simulink model "Simulation_2_Wall_Follower_v1"  (R2023a)
settings: Solver=ode1  StartTime=0.0  StopTime=inf  RelTol=1e-3
values from neighbouring files (symbols this model uses):
  D = [ D0 D1 D2 D3 D4 ]    [constante.m]    (also in data.mat = [8 8 8 8 8])
  K = [ K0 K1  0 K3 K4 ]    [constante.m]    (also in data.mat = [1.0471975512 0.523598775598 0 -0.523598775598 -1.0471975512)
  L = 5    [constante.m]    (also in data.mat)
  maze = gobjects    [animation.m]    (also in data.mat = [0 0 0 0 0 0 0 0 0 0 0 0 ... (94249 elements, 307x307)]; setup.m = cat(2,maze,add_column))
  number_add = 50    [data.mat]    (also in setup.m)
  S_max = 20    [constante.m]    (also in data.mat)
  S_sens = 0.1    [constante.m]    (also in data.mat)
  size_map = 307    [data.mat]    (also in setup.m = length(maze))
  Theta_d = -1.57079632679    [data.mat]
  Vd = 0.05    [data.mat]    (also in setup.m)
  Vg = 0.05    [data.mat]    (also in setup.m)
  Xd = 70    [data.mat]
  Yd = 170    [data.mat]
settings Model: Creator=Nas  LastModifiedBy=lespi
settings SolverCC: AlgebraicLoopSolver=TrustRegion
settings DataIOCC: ReturnWorkspaceOutputs=off
settings DebuggingCC: UnconnectedInputMsg=warning  UnconnectedOutputMsg=warning  UnconnectedLineMsg=warning  ArithmeticOperatorsInVariantConditions=warning
settings ModelReferenceCC: EnableRefExpFcnMdlSchedulingChecks=on
settings SFSimCC: SimUseLocalCustomCode=off  CustomCodeUndefinedFunction=UseInterfaceOnly
settings RTWCC: RTWUseLocalCustomCode=off

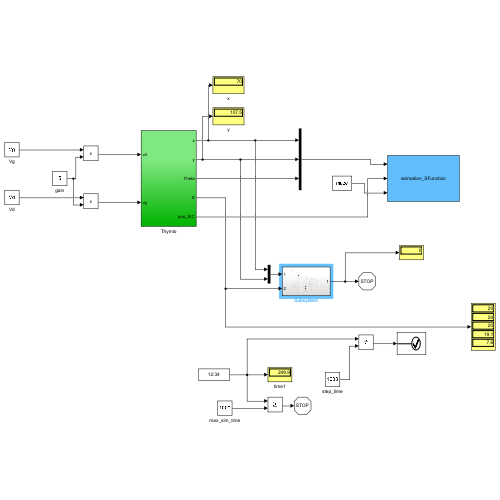
[thumbnail: Simulink's stored preview of the top-level diagram]
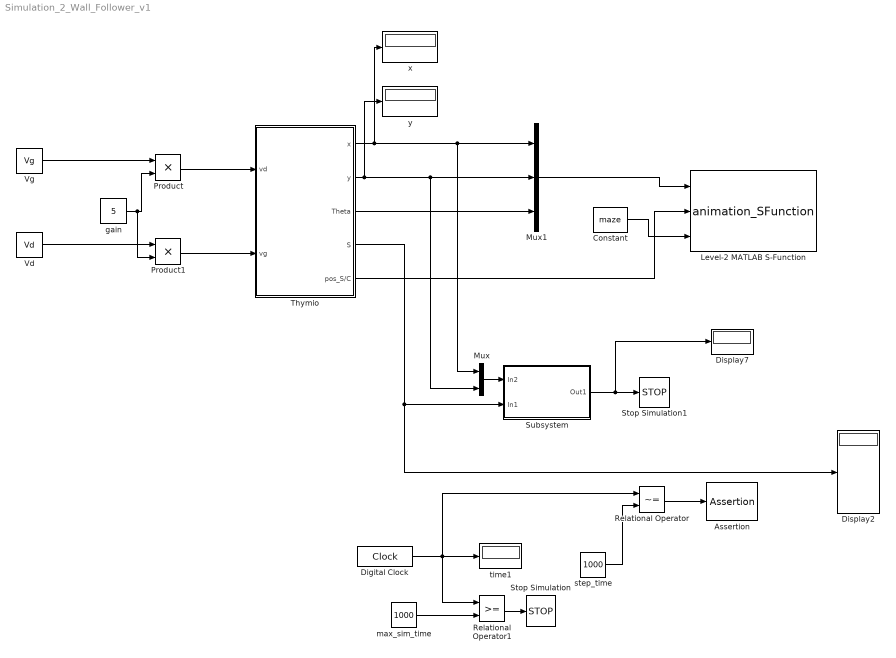
== system Simulation_2_Wall_Follower_v1 ==
  Assertion : Assertion  AssertionFailFcn=set_param(bdroot,'SimulationCommand','pause')  StopWhenAssertionFail=off
  Constant : Constant  Value=maze
  Digital Clock : DigitalClock  SampleTime=0.1
  Display2 : Display
  Display7 : Display
  Level-2 MATLAB S-Function : M-S-Function  FunctionName=animation_SFunction
  Mux : Mux  Inputs=2
  Mux1 : Mux  Inputs=3
  Product : Product
  Product1 : Product
  Relational Operator : RelationalOperator  Operator=~=  OutDataTypeStr=boolean  RndMeth=Simplest  InputSameDT=off
  Relational Operator1 : RelationalOperator  OutDataTypeStr=boolean  RndMeth=Simplest  InputSameDT=off
  Stop Simulation : Stop
  Stop Simulation1 : Stop
  Subsystem : Subsystem
  Thymio : Subsystem
  Vd : Constant  Value=Vd
  Vg : Constant  Value=Vg
  gain : Constant  Value=5
  max_sim_time : Constant  Value=1000
  step_time : Constant  Value=1000
  time1 : Display
  x : Display
  y : Display
  wires:
  Vd/1 -> Product1/1
  Vg/1 -> Product/1
  Mux1/1 -> Level-2 MATLAB S-Function/1
  Thymio/5(pos_S/C) -> Level-2 MATLAB S-Function/2
  Thymio/1(x) -> x/1, Mux/1, Mux1/1
  Mux/1 -> Subsystem/1(In2)
  Thymio/3(Theta) -> Mux1/3
  Thymio/2(y) -> Mux/2, Mux1/2, y/1
  Thymio/4(S) -> Display2/1, Subsystem/2(In1)
  Constant/1 -> Level-2 MATLAB S-Function/3
  gain/1 -> Product1/2, Product/2
  Product1/1 -> Thymio/2(vg)
  Product/1 -> Thymio/1(vd)
  step_time/1 -> Relational Operator/2
  Relational Operator/1 -> Assertion/1
  Digital Clock/1 -> time1/1, Relational Operator1/1, Relational Operator/1
  max_sim_time/1 -> Relational Operator1/2
  Relational Operator1/1 -> Stop Simulation/1
  Subsystem/1(Out1) -> Display7/1, Stop Simulation1/1

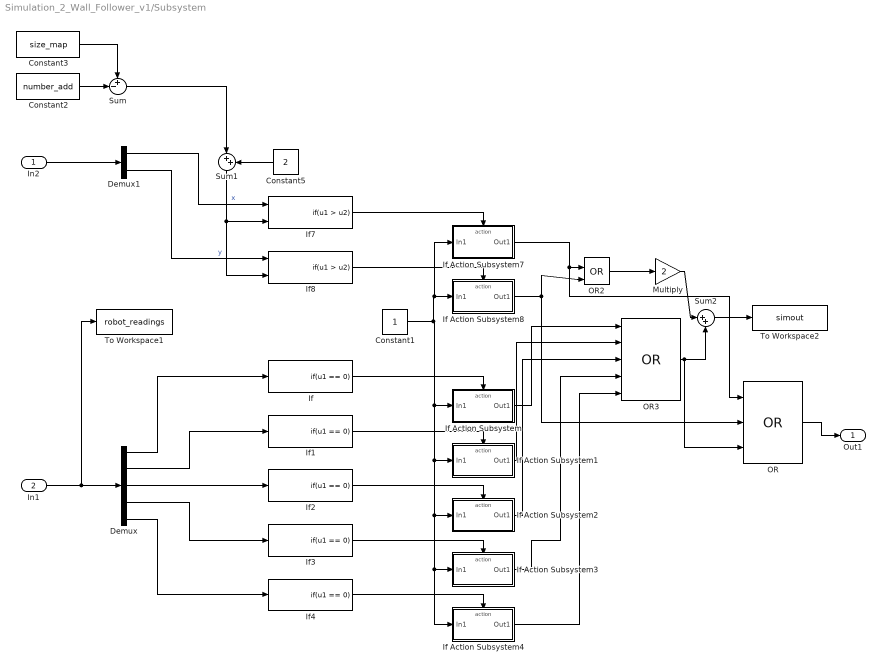
== system Simulation_2_Wall_Follower_v1/Subsystem ==
  In2 : Inport
  In1 : Inport  Port=2
  Constant1 : Constant
  Constant2 : Constant  Value=number_add
  Constant3 : Constant  Value=size_map
  Constant5 : Constant  Value=2
  Demux : Demux  Outputs=5
  Demux1 : Demux  Outputs=2
  If{,1..4} (5 alike) : If  IfExpression=u1 == 0  ShowElse=off
  If Action Subsystem : Subsystem  TreatAsAtomicUnit=on
  If Action Subsystem1 : Subsystem  TreatAsAtomicUnit=on
  If Action Subsystem2 : Subsystem  TreatAsAtomicUnit=on
  If Action Subsystem3 : Subsystem  TreatAsAtomicUnit=on
  If Action Subsystem4 : Subsystem  TreatAsAtomicUnit=on
  If Action Subsystem7 : Subsystem  TreatAsAtomicUnit=on
  If Action Subsystem8 : Subsystem  TreatAsAtomicUnit=on
  If7 : If  NumInputs=2  IfExpression=u1 > u2  ShowElse=off
  If8 : If  NumInputs=2  IfExpression=u1 > u2  ShowElse=off
  Multiply : Gain  Gain=2
  OR : Logic  Operator=OR  Inputs=3  IconShape=distinctive  AllPortsSameDT=off  OutDataTypeStr=boolean
  OR2 : Logic  Operator=OR  IconShape=distinctive  AllPortsSameDT=off  OutDataTypeStr=boolean
  OR3 : Logic  Operator=OR  Inputs=5  IconShape=distinctive  AllPortsSameDT=off  OutDataTypeStr=boolean
  Sum : Sum  Inputs=+-|
  Sum1 : Sum  Inputs=|++
  Sum2 : Sum  Inputs=|++
  To Workspace1 : ToWorkspace  VariableName=robot_readings  SaveFormat=Timeseries  SampleTime=-1
      settings: MaxDataPoints=1
  To Workspace2 : ToWorkspace  VariableName=simout  SaveFormat=Timeseries  SampleTime=-1
      settings: MaxDataPoints=1
  Out1 : Outport  VectorParamsAs1DForOutWhenUnconnected=off
  wires:
  Constant1/1 -> If Action Subsystem7/1(In1), If Action Subsystem8/1(In1), If Action Subsystem1/1(In1), If Action Subsystem2/1(In1), If Action Subsystem3/1(In1), If Action Subsystem4/1(In1), If Action Subsystem/1(In1)
  In1/1 -> To Workspace1/1, Demux/1
  Demux/1 -> If/1
  Demux/2 -> If1/1
  Demux/3 -> If2/1
  Demux/4 -> If3/1
  Demux/5 -> If4/1
  If/1 -> If Action Subsystem/Action
  If1/1 -> If Action Subsystem1/Action
  If2/1 -> If Action Subsystem2/Action
  If3/1 -> If Action Subsystem3/Action
  If4/1 -> If Action Subsystem4/Action
  OR/1 -> Out1/1
  In2/1 -> Demux1/1
  Demux1/2 -> If8/1  "y"
  Demux1/1 -> If7/1  "x"
  Constant3/1 -> Sum/1
  Constant2/1 -> Sum/2
  Sum/1 -> Sum1/1
  Sum1/1 -> If7/2, If8/2
  Constant5/1 -> Sum1/2
  If Action Subsystem7/1(Out1) -> OR2/1, OR/1
  If Action Subsystem8/1(Out1) -> OR/2, OR2/2
  If8/1 -> If Action Subsystem8/Action
  If7/1 -> If Action Subsystem7/Action
  If Action Subsystem4/1(Out1) -> OR3/5
  If Action Subsystem3/1(Out1) -> OR3/4
  If Action Subsystem2/1(Out1) -> OR3/3
  If Action Subsystem1/1(Out1) -> OR3/2
  If Action Subsystem/1(Out1) -> OR3/1
  OR2/1 -> Multiply/1
  OR3/1 -> OR/3, Sum2/2
  Multiply/1 -> Sum2/1
  Sum2/1 -> To Workspace2/1

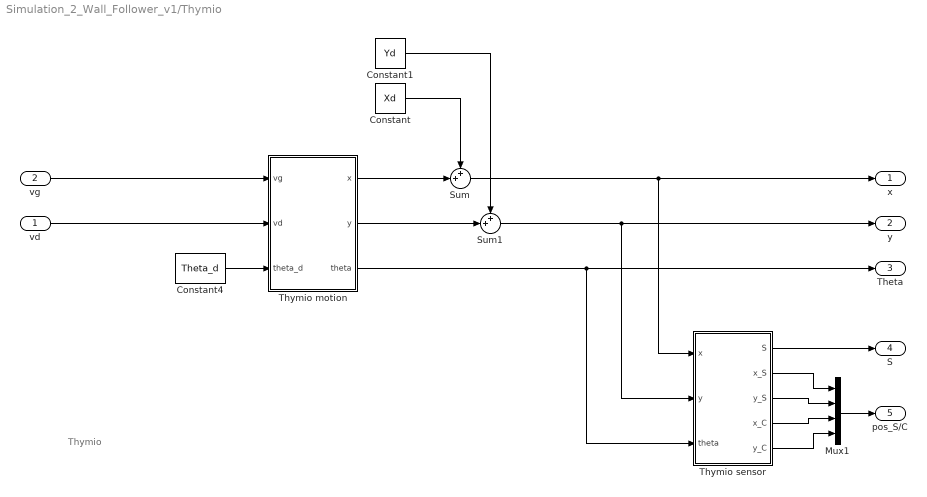
== system Simulation_2_Wall_Follower_v1/Thymio ==
  note: Thymio
  vd : Inport
  vg : Inport  Port=2
  Constant : Constant  Value=Xd
  Constant1 : Constant  Value=Yd
  Constant4 : Constant  Value=Theta_d
  Mux1 : Mux
  Sum : Sum  Inputs=++|
  Sum1 : Sum  Inputs=++|
  Thymio motion : Subsystem
  Thymio sensor : Subsystem
  x : Outport  VectorParamsAs1DForOutWhenUnconnected=off
  y : Outport  Port=2  VectorParamsAs1DForOutWhenUnconnected=off
  Theta : Outport  Port=3  VectorParamsAs1DForOutWhenUnconnected=off
  S : Outport  Port=4  VectorParamsAs1DForOutWhenUnconnected=off
  pos_S/C : Outport  Port=5  VectorParamsAs1DForOutWhenUnconnected=off
  wires:
  Constant4/1 -> Thymio motion/3(theta_d)
  Sum1/1 -> Thymio sensor/2(y), y/1
  Thymio motion/2(y) -> Sum1/2
  Constant/1 -> Sum/1
  Thymio motion/3(theta) -> Thymio sensor/3(theta), Theta/1
  Constant1/1 -> Sum1/1
  Sum/1 -> Thymio sensor/1(x), x/1
  Thymio motion/1(x) -> Sum/2
  vg/1 -> Thymio motion/1(vg)
  vd/1 -> Thymio motion/2(vd)
  Thymio sensor/1(S) -> S/1
  Thymio sensor/2(x_S) -> Mux1/1
  Thymio sensor/3(y_S) -> Mux1/2
  Mux1/1 -> pos_S/C/1
  Thymio sensor/4(x_C) -> Mux1/3
  Thymio sensor/5(y_C) -> Mux1/4

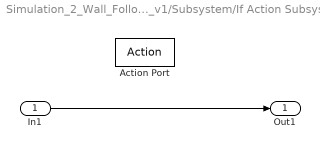
== system Simulation_2_Wall_Follower_v1/Subsystem/If Action Subsystem ==
  In1 : Inport
  Action Port : ActionPort  ActionPortLabel=if(u1 == 0)
  Out1 : Outport  VectorParamsAs1DForOutWhenUnconnected=off
  wires:
  In1/1 -> Out1/1

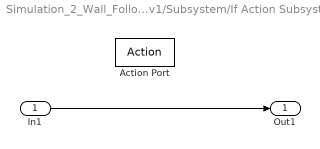
== system Simulation_2_Wall_Follower_v1/Subsystem/If Action Subsystem1 ==
  In1 : Inport
  Action Port : ActionPort  ActionPortLabel=if(u1 == 0)
  Out1 : Outport  VectorParamsAs1DForOutWhenUnconnected=off
  wires:
  In1/1 -> Out1/1

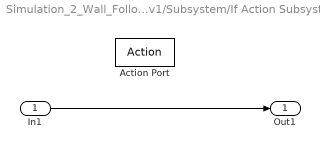
== system Simulation_2_Wall_Follower_v1/Subsystem/If Action Subsystem2 ==
  In1 : Inport
  Action Port : ActionPort  ActionPortLabel=if(u1 == 0)
  Out1 : Outport  VectorParamsAs1DForOutWhenUnconnected=off
  wires:
  In1/1 -> Out1/1

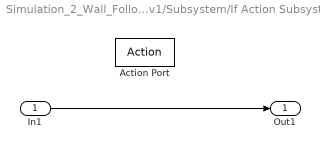
== system Simulation_2_Wall_Follower_v1/Subsystem/If Action Subsystem3 ==
  In1 : Inport
  Action Port : ActionPort  ActionPortLabel=if(u1 == 0)
  Out1 : Outport  VectorParamsAs1DForOutWhenUnconnected=off
  wires:
  In1/1 -> Out1/1

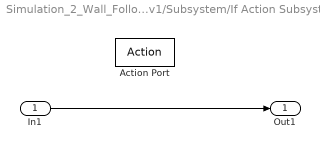
== system Simulation_2_Wall_Follower_v1/Subsystem/If Action Subsystem4 ==
  In1 : Inport
  Action Port : ActionPort  ActionPortLabel=if(u1 == 0)
  Out1 : Outport  VectorParamsAs1DForOutWhenUnconnected=off
  wires:
  In1/1 -> Out1/1

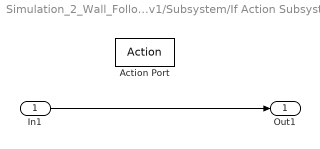
== system Simulation_2_Wall_Follower_v1/Subsystem/If Action Subsystem7 ==
  In1 : Inport
  Action Port : ActionPort  ActionPortLabel=if(u1 > u2)
  Out1 : Outport  VectorParamsAs1DForOutWhenUnconnected=off
  wires:
  In1/1 -> Out1/1

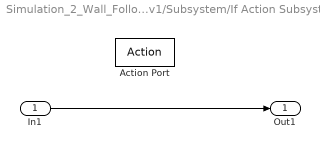
== system Simulation_2_Wall_Follower_v1/Subsystem/If Action Subsystem8 ==
  In1 : Inport
  Action Port : ActionPort  ActionPortLabel=if(u1 > u2)
  Out1 : Outport  VectorParamsAs1DForOutWhenUnconnected=off
  wires:
  In1/1 -> Out1/1

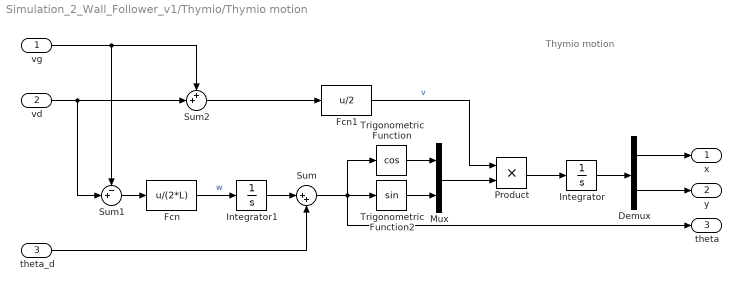
== system Simulation_2_Wall_Follower_v1/Thymio/Thymio motion ==
  note: Thymio motion
  vg : Inport
  vd : Inport  Port=2
  theta_d : Inport  Port=3
  Demux : Demux  Outputs=2
  Fcn : Fcn  Expr=u/(2*L)
  Fcn1 : Fcn  Expr=u/2
  Integrator : Integrator
  Integrator1 : Integrator
  Mux : Mux  Inputs=2
  Product : Product  RndMeth=Zero
  Sum : Sum  Inputs=|++
  Sum1 : Sum  Inputs=-+|
  Sum2 : Sum  Inputs=++|
  Trigonometric Function : Trigonometry  Operator=cos
  Trigonometric Function2 : Trigonometry
  x : Outport  VectorParamsAs1DForOutWhenUnconnected=off
  y : Outport  Port=2  VectorParamsAs1DForOutWhenUnconnected=off
  theta : Outport  Port=3  VectorParamsAs1DForOutWhenUnconnected=off
  wires:
  Sum/1 -> theta/1, Trigonometric Function/1, Trigonometric Function2/1
  vd/1 -> Sum2/2, Sum1/2
  vg/1 -> Sum2/1, Sum1/1
  Sum1/1 -> Fcn/1
  Fcn/1 -> Integrator1/1  "w"
  Sum2/1 -> Fcn1/1
  Demux/2 -> y/1
  Demux/1 -> x/1
  Fcn1/1 -> Product/1  "v"
  Product/1 -> Integrator/1
  Mux/1 -> Product/2
  Integrator/1 -> Demux/1
  Trigonometric Function2/1 -> Mux/2
  Trigonometric Function/1 -> Mux/1
  Integrator1/1 -> Sum/1
  theta_d/1 -> Sum/2

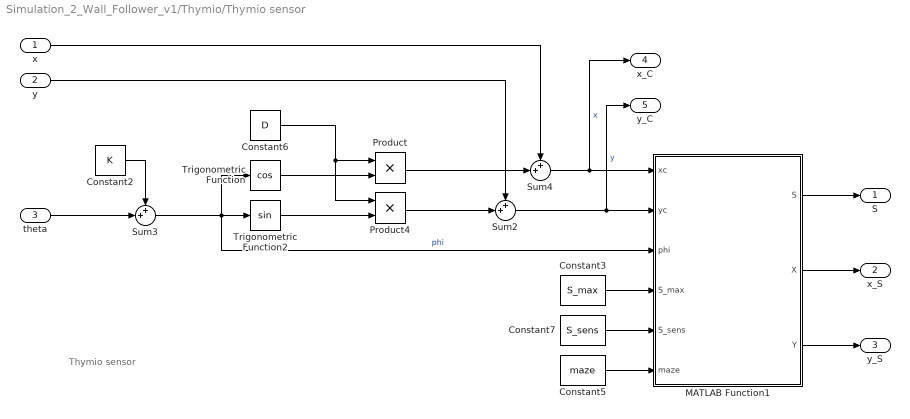
== system Simulation_2_Wall_Follower_v1/Thymio/Thymio sensor ==
  note: Thymio sensor
  x : Inport
  y : Inport  Port=2
  theta : Inport  Port=3
  Constant2 : Constant  Value=K
  Constant3 : Constant  Value=S_max
  Constant5 : Constant  Value=maze  VectorParams1D=off
  Constant6 : Constant  Value=D
  Constant7 : Constant  Value=S_sens
  MATLAB Function1 : MATLAB Function  TreatAsAtomicUnit=on
  Product : Product
  Product4 : Product
  Sum2 : Sum  Inputs=++|
  Sum3 : Sum  Inputs=++|
  Sum4 : Sum  Inputs=++|
  Trigonometric Function : Trigonometry  Operator=cos
  Trigonometric Function2 : Trigonometry
  S : Outport  VectorParamsAs1DForOutWhenUnconnected=off
  x_S : Outport  Port=2  VectorParamsAs1DForOutWhenUnconnected=off
  y_S : Outport  Port=3  VectorParamsAs1DForOutWhenUnconnected=off
  x_C : Outport  Port=4  VectorParamsAs1DForOutWhenUnconnected=off
  y_C : Outport  Port=5  VectorParamsAs1DForOutWhenUnconnected=off
  wires:
  y/1 -> Sum2/1
  Constant5/1 -> MATLAB Function1/6(maze)
  Constant2/1 -> Sum3/1
  Trigonometric Function/1 -> Product/2
  theta/1 -> Sum3/2
  Constant6/1 -> Product4/1, Product/1
  Sum2/1 -> y_C/1, MATLAB Function1/2(yc)  "y"
  MATLAB Function1/2(X) -> x_S/1
  x/1 -> Sum4/1
  Product4/1 -> Sum2/2
  Constant3/1 -> MATLAB Function1/4(S_max)
  Sum4/1 -> x_C/1, MATLAB Function1/1(xc)  "x"
  Sum3/1 -> Trigonometric Function/1, MATLAB Function1/3(phi), Trigonometric Function2/1  "phi"
  MATLAB Function1/1(S) -> S/1
  MATLAB Function1/3(Y) -> y_S/1
  Trigonometric Function2/1 -> Product4/2
  Constant7/1 -> MATLAB Function1/5(S_sens)
  Product/1 -> Sum4/2

== matlab function Simulation_2_Wall_Follower_v1/Thymio/Thymio sensor/MATLAB Function1 ==
  data: xc input; S output; yc input; phi input; S_max input; S_sens input; maze input; X output; Y output
%% %%%%%%%%%%%%%%%%%%%%%%%%%%%%%%%%%%%%%%%%%%%%%%%%%%%%%%%%%%%%%%%%%%%%%
%%  [S,X,Y] = sensor_value(xc, yc, phi, S_max, S_sens, maze)
%% %%%%%%%%%%%%%%%%%%%%%%%%%%%%%%%%%%%%%%%%%%%%%%%%%%%%%%%%%%%%%%%%%%%%%
%% Description : Computes the distance between a wall and each sensor
%%               until a given limit.
%%
%% Input : xc (vector) = Coordinate of each sensor on the x-axe
%%         yc (vector) = Coordinate of each sensor on the y-axe
%%         phi (vector) = Angular coordinate of each sensor
%%         S_max (scalar) = Maximum range of sensors
%%         S_sens (scalar) = Sensors sensibility
%%         maze (matrice) = Picture of the maze
%%
%% Output : S (vector) = Signal of each sensor with :
%%                            S = S_max  ->  no wall
%%                            S < S_max  ->  détected wall
%%          X (vector) = Position of the signal S in the x-axe to his
%%                         sensor
%%          Y (vector) = Position of the signal S in the y-axe to his
%%                         sensor
%%
%% Date : 28/03/2018
%% Release : 2.0
%% %%%%%%%%%%%%%%%%%%%%%%%%%%%%%%%%%%%%%%%%%%%%%%%%%%%%%%%%%%%%%%%%%%%%%



function [S,X,Y] = sensor_value(xc, yc, phi, S_max, S_sens, maze)

  Nb_capteur = length(xc);

  % Initialization
  S = zeros(Nb_capteur,1);
  X = zeros(Nb_capteur,1);
  Y = zeros(Nb_capteur,1);

  for capteur = 1:1:Nb_capteur
    for signal = 0:S_sens:S_max

      dx = signal * cos(phi(capteur));
      dy = signal * sin(phi(capteur));

      % Set the next position to test
      X(capteur) = xc(capteur) + dx;
      Y(capteur) = yc(capteur) + dy;

      % Test if a wall is present
      if maze(round(Y(capteur)),round(X(capteur))) == 1

        S(capteur) = sqrt(dx^2 + dy^2);
        break      % Stop the for loop
          
      else
        S(capteur) = signal;
        
      end

    end
  end
  
  
end



%% %%%%%%%%%%%%%%%%%%%%%%%%%%%%%%%%%%%%%%%%%%%%%%%%%%%%%%%%%%%%%%%%%%%%%%
